simulink model "DOE_MODEL_4D"  (R2017a)
settings: Solver=VariableStepAuto  StartTime=0.0  StopTime=100  RelTol=1e-3
libraries: simulink x2
settings Model: Creator=HP  LastModifiedBy=jianx

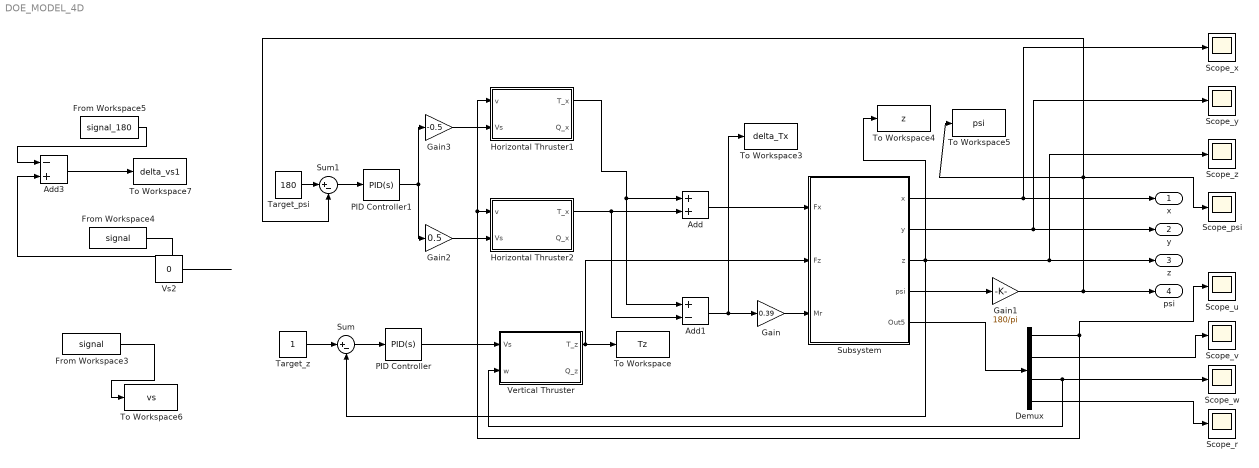
== system DOE_MODEL_4D ==
  Add : Sum
  Add1 : Sum  Inputs=+-
  Add3 : Sum  Inputs=-+
  Demux : Demux
  From Workspace3 : FromWorkspace  VariableName=signal  OutputAfterFinalValue=Setting to zero
  From Workspace4 : FromWorkspace  VariableName=signal  OutputAfterFinalValue=Setting to zero
  From Workspace5 : FromWorkspace  VariableName=signal_180  OutputAfterFinalValue=Setting to zero
  Gain : Gain  Gain=0.39
  Gain1 : Gain  Gain=180/pi
  Gain2 : Gain  Gain=0.5
  Gain3 : Gain  Gain=-0.5
  Horizontal Thruster1 : Subsystem
  Horizontal Thruster2 : Subsystem
  PID Controller : simulink/Continuous/PID Controller  Controller=PID  TimeDomain=Continuous-time  SampleTime=-1  IntegratorMethod=Forward Euler  FilterMethod=Forward Euler  Form=Parallel  UseFilter=on  ControllerParametersSource=internal  P=200  I=11.6  D=872.4  N=100  InitialConditionSource=internal  InitialConditionForIntegrator=0  InitialConditionForFilter=0  ExternalReset=none  LimitOutput=off  UpperSaturationLimit=inf  LowerSaturationLimit=-inf  LinearizeAsGain=on  AntiWindupMode=none  Kb=1  TrackingMode=off  Kt=1  PParamMin=[]  PParamMax=[]  IParamMin=[]  IParamMax=[]  DParamMin=[]  DParamMax=[]  NParamMin=[]  NParamMax=[]  KbParamMin=[]  KbParamMax=[]  KtParamMin=[]  KtParamMax=[]  POutMin=[]  POutMax=[]  IOutMin=[]  IOutMax=[]  DOutMin=[]  DOutMax=[]  NOutMin=[]  NOutMax=[]  KbOutMin=[]  KbOutMax=[]  KtOutMin=[]  KtOutMax=[]  IntegratorOutMin=[]  IntegratorOutMax=[]  FilterOutMin=[]  FilterOutMax=[]  SumOutMin=[]  SumOutMax=[]  SumI1OutMin=[]  SumI1OutMax=[]  SumI2OutMin=[]  SumI2OutMax=[]  SumI3OutMin=[]  SumI3OutMax=[]  SumDOutMin=[]  SumDOutMax=[]  SaturationOutMin=[]  SaturationOutMax=[]  IntegratorContinuousStateAttributes=''  IntegratorStateMustResolveToSignalObject=off  IntegratorRTWStateStorageClass=Auto  FilterContinuousStateAttributes=''  FilterStateMustResolveToSignalObject=off  FilterRTWStateStorageClass=Auto  DifferentiatorICPrevScaledInput=0  DifferentiatorOutMin=[]  DifferentiatorOutMax=[]  InitialConditionSetting=State (most efficient)
  PID Controller1 : simulink/Continuous/PID Controller  Controller=PID  TimeDomain=Continuous-time  SampleTime=-1  IntegratorMethod=Forward Euler  FilterMethod=Forward Euler  Form=Parallel  UseFilter=on  ControllerParametersSource=internal  P=-0.57  I=-0.021  D=-0.918  N=100  InitialConditionSource=internal  InitialConditionForIntegrator=0  InitialConditionForFilter=0  ExternalReset=none  LimitOutput=off  UpperSaturationLimit=inf  LowerSaturationLimit=-inf  LinearizeAsGain=on  AntiWindupMode=none  Kb=1  TrackingMode=off  Kt=1  PParamMin=[]  PParamMax=[]  IParamMin=[]  IParamMax=[]  DParamMin=[]  DParamMax=[]  NParamMin=[]  NParamMax=[]  KbParamMin=[]  KbParamMax=[]  KtParamMin=[]  KtParamMax=[]  POutMin=[]  POutMax=[]  IOutMin=[]  IOutMax=[]  DOutMin=[]  DOutMax=[]  NOutMin=[]  NOutMax=[]  KbOutMin=[]  KbOutMax=[]  KtOutMin=[]  KtOutMax=[]  IntegratorOutMin=[]  IntegratorOutMax=[]  FilterOutMin=[]  FilterOutMax=[]  SumOutMin=[]  SumOutMax=[]  SumI1OutMin=[]  SumI1OutMax=[]  SumI2OutMin=[]  SumI2OutMax=[]  SumI3OutMin=[]  SumI3OutMax=[]  SumDOutMin=[]  SumDOutMax=[]  SaturationOutMin=[]  SaturationOutMax=[]  IntegratorContinuousStateAttributes=''  IntegratorStateMustResolveToSignalObject=off  IntegratorRTWStateStorageClass=Auto  FilterContinuousStateAttributes=''  FilterStateMustResolveToSignalObject=off  FilterRTWStateStorageClass=Auto  DifferentiatorICPrevScaledInput=0  DifferentiatorOutMin=[]  DifferentiatorOutMax=[]  InitialConditionSetting=State (most efficient)
  Scope_psi : Scope
  Scope_r : Scope
  Scope_u : Scope
  Scope_v : Scope
  Scope_w : Scope
  Scope_x : Scope
  Scope_y : Scope
  Scope_z : Scope
  Subsystem : Subsystem
  Sum : Sum  Inputs=|+-
  Sum1 : Sum  Inputs=|+-
  Target_psi : Constant  Value=180
  Target_z : Constant
  To Workspace : ToWorkspace  VariableName=Tz  SampleTime=[0.002,0]
  To Workspace3 : ToWorkspace  VariableName=delta_Tx  SampleTime=[0.002,0]
  To Workspace4 : ToWorkspace  VariableName=z  SampleTime=[0.002,0]
  To Workspace5 : ToWorkspace  VariableName=psi  SampleTime=[0.002,0]
  To Workspace6 : ToWorkspace  VariableName=vs  SampleTime=0.002
      settings: Save2DSignal=2-D array (concatenate along first dimension)
  To Workspace7 : ToWorkspace  VariableName=delta_vs1  SampleTime=0.002
      settings: Save2DSignal=2-D array (concatenate along first dimension)
  "Vertical Thruster " : Subsystem
  Vs2 : Constant  Value=0
  x : Outport
  y : Outport  Port=2
  z : Outport  Port=3
  psi : Outport  Port=4
  wires:
  Add/1 -> Subsystem/1(Fx)
  "Vertical Thruster "/1(T_z) -> Subsystem/2(Fz), To Workspace/1
  Add1/1 -> To Workspace3/1, Gain/1
  Subsystem/1(x) -> Scope_x/1, x/1
  Subsystem/2(y) -> y/1, Scope_y/1
  Subsystem/4(psi) -> Gain1/1
  Subsystem/3(z) -> Sum/2, To Workspace4/1, z/1, Scope_z/1
  Subsystem/5(Out5) -> Demux/1
  Demux/3 -> Scope_w/1, "Vertical Thruster "/2(w)
  Demux/1 -> Horizontal Thruster1/1(v), Horizontal Thruster2/1(v), Scope_u/1
  Horizontal Thruster1/1(T_x) -> Add1/1, Add/1
  Horizontal Thruster2/1(T_x) -> Add1/2, Add/2
  Gain/1 -> Subsystem/3(Mr)
  Demux/2 -> Scope_v/1
  Gain1/1 -> Sum1/2, To Workspace5/1, Scope_psi/1, psi/1
  Demux/4 -> Scope_r/1
  From Workspace3/1 -> To Workspace6/1
  From Workspace5/1 -> Add3/1
  Add3/1 -> To Workspace7/1
  From Workspace4/1 -> Add3/2
  Vs2/1 -> ?
  Sum/1 -> PID Controller/1
  PID Controller1/1 -> Gain2/1, Gain3/1
  Sum1/1 -> PID Controller1/1
  Target_z/1 -> Sum/1
  Target_psi/1 -> Sum1/1
  Gain3/1 -> Horizontal Thruster1/2(Vs)
  Gain2/1 -> Horizontal Thruster2/2(Vs)
  PID Controller/1 -> "Vertical Thruster "/1(Vs)

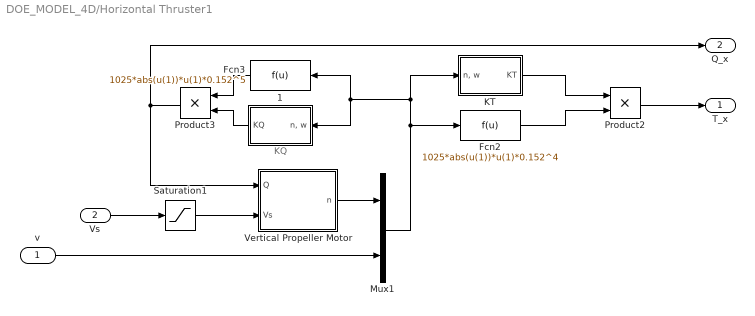
== system DOE_MODEL_4D/Horizontal Thruster1 ==
  note: KQ
  v : Inport
  Vs : Inport  Port=2
  " 1" : Subsystem
  " Vertical Propeller Motor " : Subsystem
  Fcn2 : Fcn  Expr=1025*abs(u(1))*u(1)*0.152^4
  Fcn3 : Fcn  Expr=1025*abs(u(1))*u(1)*0.152^5
  KT : Subsystem
  Mux1 : Mux  Inputs=2
  Product2 : Product
  Product3 : Product
  Saturation1 : Saturate  UpperLimit=100  LowerLimit=-100
  T_x : Outport
  Q_x : Outport  Port=2
  wires:
  Mux1/1 -> KT/1("n, w"), " 1"/1("n, w"), Fcn3/1, Fcn2/1
  Fcn3/1 -> Product3/1
  Product3/1 -> " Vertical Propeller Motor "/1("Q "), Q_x/1
  v/1 -> Mux1/2
  Fcn2/1 -> Product2/2
  " Vertical Propeller Motor "/1(n) -> Mux1/1
  KT/1(KT) -> Product2/1
  " 1"/1(KQ) -> Product3/2
  Saturation1/1 -> " Vertical Propeller Motor "/2(Vs)
  Vs/1 -> Saturation1/1
  Product2/1 -> T_x/1

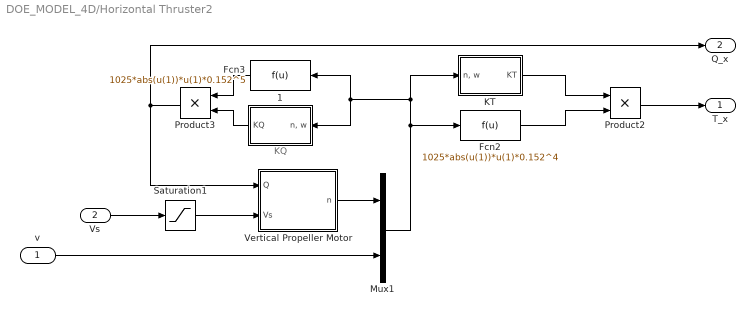
== system DOE_MODEL_4D/Horizontal Thruster2 ==
  note: KQ
  v : Inport
  Vs : Inport  Port=2
  " 1" : Subsystem
  " Vertical Propeller Motor " : Subsystem
  Fcn2 : Fcn  Expr=1025*abs(u(1))*u(1)*0.152^4
  Fcn3 : Fcn  Expr=1025*abs(u(1))*u(1)*0.152^5
  KT : Subsystem
  Mux1 : Mux  Inputs=2
  Product2 : Product
  Product3 : Product
  Saturation1 : Saturate  UpperLimit=100  LowerLimit=-100
  T_x : Outport
  Q_x : Outport  Port=2
  wires:
  Mux1/1 -> KT/1("n, w"), " 1"/1("n, w"), Fcn3/1, Fcn2/1
  Fcn3/1 -> Product3/1
  Product3/1 -> " Vertical Propeller Motor "/1("Q "), Q_x/1
  v/1 -> Mux1/2
  Fcn2/1 -> Product2/2
  " Vertical Propeller Motor "/1(n) -> Mux1/1
  KT/1(KT) -> Product2/1
  " 1"/1(KQ) -> Product3/2
  Saturation1/1 -> " Vertical Propeller Motor "/2(Vs)
  Vs/1 -> Saturation1/1
  Product2/1 -> T_x/1

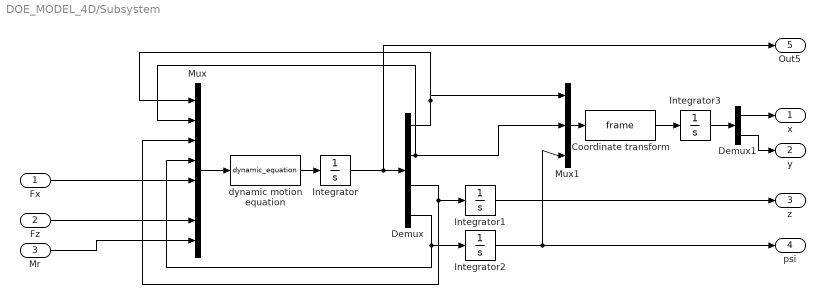
== system DOE_MODEL_4D/Subsystem ==
  Fx : Inport
  Fz : Inport  Port=2
  Mr : Inport  Port=3
  "Coordinate transform " : MATLABFcn  MATLABFcn=frame  OutputDimensions=2
  Demux : Demux
  Demux1 : Demux  Outputs=2
  Integrator{,1..3} (4 alike) : Integrator
  Mux : Mux  Inputs=8
  Mux1 : Mux  Inputs=3
  "dynamic motion equation " : MATLABFcn  MATLABFcn=dynamic_equation  OutputDimensions=4
  x : Outport
  y : Outport  Port=2
  z : Outport  Port=3
  psi : Outport  Port=4
  Out5 : Outport  Port=5
  wires:
  Fz/1 -> Mux/7
  Demux/1 -> Mux1/1, Mux/1
  Mr/1 -> Mux/8
  Integrator/1 -> Out5/1, Demux/1
  Demux/2 -> Mux1/2, Mux/2
  Demux/4 -> Integrator2/1, Mux/4
  Mux/1 -> "dynamic motion equation "/1
  Fx/1 -> Mux/5
  "dynamic motion equation "/1 -> Integrator/1
  Demux/3 -> Integrator1/1, Mux/3
  Mux1/1 -> "Coordinate transform "/1
  Integrator2/1 -> psi/1, Mux1/3
  Integrator1/1 -> z/1
  "Coordinate transform "/1 -> Integrator3/1
  Demux1/1 -> x/1
  Demux1/2 -> y/1
  Integrator3/1 -> Demux1/1

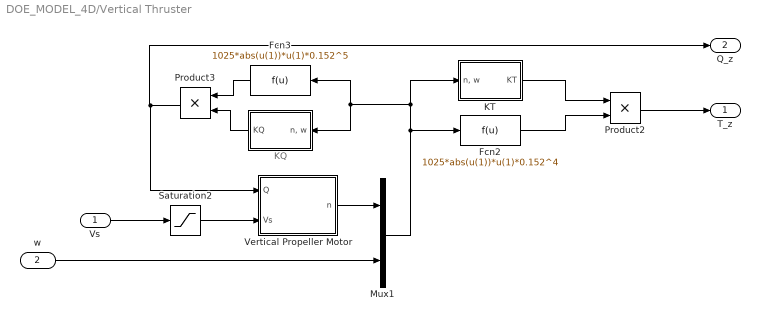
== system DOE_MODEL_4D/Vertical Thruster  ==
  note: KQ
  Vs : Inport
  w : Inport  Port=2
  " " : Subsystem
  " Vertical Propeller Motor " : Subsystem
  Fcn2 : Fcn  Expr=1025*abs(u(1))*u(1)*0.152^4
  Fcn3 : Fcn  Expr=1025*abs(u(1))*u(1)*0.152^5
  KT : Subsystem
  Mux1 : Mux  Inputs=2
  Product2 : Product
  Product3 : Product
  Saturation2 : Saturate  UpperLimit=100  LowerLimit=-100
  T_z : Outport
  Q_z : Outport  Port=2
  wires:
  Mux1/1 -> KT/1("n, w"), " "/1("n, w"), Fcn3/1, Fcn2/1
  Product2/1 -> T_z/1
  Fcn3/1 -> Product3/1
  Product3/1 -> " Vertical Propeller Motor "/1("Q "), Q_z/1
  w/1 -> Mux1/2
  Fcn2/1 -> Product2/2
  " Vertical Propeller Motor "/1(n) -> Mux1/1
  KT/1(KT) -> Product2/1
  " "/1(KQ) -> Product3/2
  Saturation2/1 -> " Vertical Propeller Motor "/2(Vs)
  Vs/1 -> Saturation2/1

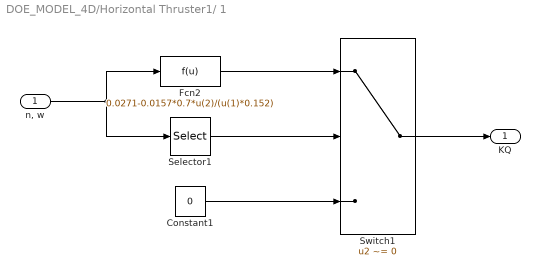
== system DOE_MODEL_4D/Horizontal Thruster1/ 1 ==
  "n, w" : Inport
  Constant1 : Constant  Value=0
  Fcn2 : Fcn  Expr=0.0271-0.0157*0.7*u(2)/(u(1)*0.152)
  Selector1 : Selector  InputPortWidth=2  IndexOptions=Index vector (dialog)  Indices=[ 1 ]  OutputSizes=1
  Switch1 : Switch  Criteria=u2 ~= 0
  KQ : Outport
  wires:
  Constant1/1 -> Switch1/3
  Switch1/1 -> KQ/1
  Fcn2/1 -> Switch1/1
  "n, w"/1 -> Fcn2/1, Selector1/1
  Selector1/1 -> Switch1/2

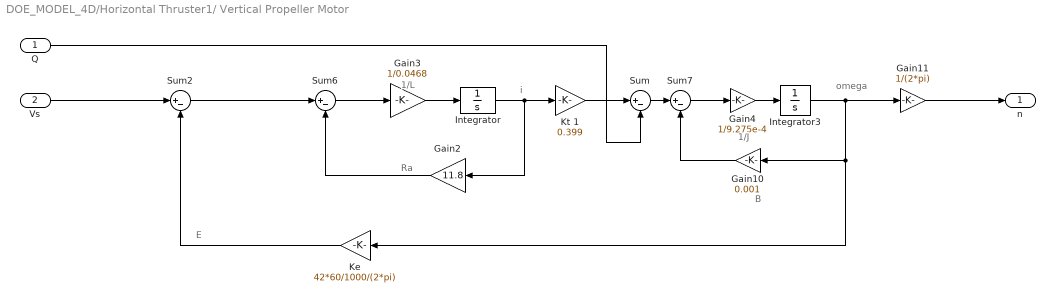
== system DOE_MODEL_4D/Horizontal Thruster1/ Vertical Propeller Motor  ==
  note: Ra
  note: i
  note: 1/J
  note: 1/L
  note: B
  note: omega
  note: E
  "Q " : Inport
  Vs : Inport  Port=2
  Gain10 : Gain  Gain=0.001  SaturateOnIntegerOverflow=on  OutDataTypeStr=Inherit: Same as input  ParamDataTypeStr=Inherit: Same as input
  Gain11 : Gain  Gain=1/(2*pi)  SaturateOnIntegerOverflow=on  OutDataTypeStr=Inherit: Same as input  ParamDataTypeStr=Inherit: Same as input
  Gain2 : Gain  Gain=11.8  OutDataTypeStr=Inherit: Same as input  ParamDataTypeStr=Inherit: Same as input
  Gain3 : Gain  Gain=1/0.0468  OutDataTypeStr=Inherit: Same as input  ParamDataTypeStr=Inherit: Same as input
  Gain4 : Gain  Gain=1/9.275e-4  SaturateOnIntegerOverflow=on  OutDataTypeStr=Inherit: Same as input  ParamDataTypeStr=Inherit: Same as input
  Integrator : Integrator
  Integrator3 : Integrator
  Ke : Gain  Gain=42*60/1000/(2*pi)
  Kt 1 : Gain  Gain=0.399
  Sum : Sum  Inputs=|+-
  Sum2 : Sum  Inputs=|+-  SaturateOnIntegerOverflow=on  InputSameDT=on  OutDataTypeStr=Inherit: Same as first input
  Sum6 : Sum  Inputs=|+-  SaturateOnIntegerOverflow=on  InputSameDT=on  OutDataTypeStr=Inherit: Same as first input
  Sum7 : Sum  Inputs=|+-  SaturateOnIntegerOverflow=on  InputSameDT=on  OutDataTypeStr=Inherit: Same as first input
  n : Outport
  wires:
  "Q "/1 -> Sum/2
  Kt 1/1 -> Sum/1
  Vs/1 -> Sum2/1
  Sum/1 -> Sum7/1
  Sum7/1 -> Gain4/1
  Gain4/1 -> Integrator3/1
  Integrator3/1 -> Ke/1, Gain10/1, Gain11/1
  Gain10/1 -> Sum7/2
  Sum2/1 -> Sum6/1
  Gain3/1 -> Integrator/1
  Gain2/1 -> Sum6/2
  Sum6/1 -> Gain3/1
  Integrator/1 -> Gain2/1, Kt 1/1
  Ke/1 -> Sum2/2
  Gain11/1 -> n/1

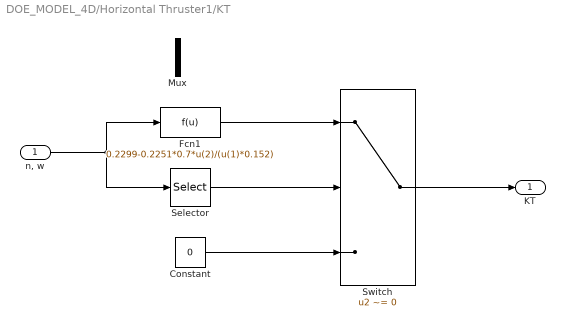
== system DOE_MODEL_4D/Horizontal Thruster1/KT ==
  "n, w" : Inport
  Constant : Constant  Value=0
  Fcn1 : Fcn  Expr=0.2299-0.2251*0.7*u(2)/(u(1)*0.152)
  Mux : Mux  Inputs=2
  Selector : Selector  InputPortWidth=2  IndexOptions=Index vector (dialog)  Indices=[ 1 ]  OutputSizes=1
  Switch : Switch  Criteria=u2 ~= 0
  KT : Outport
  wires:
  Switch/1 -> KT/1
  Constant/1 -> Switch/3
  Fcn1/1 -> Switch/1
  Selector/1 -> Switch/2
  "n, w"/1 -> Fcn1/1, Selector/1

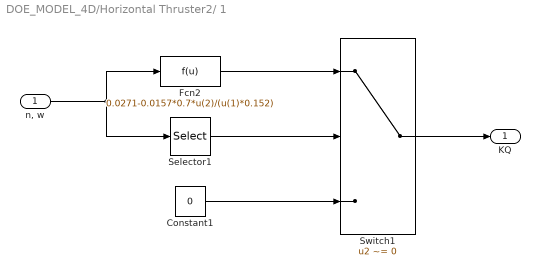
== system DOE_MODEL_4D/Horizontal Thruster2/ 1 ==
  "n, w" : Inport
  Constant1 : Constant  Value=0
  Fcn2 : Fcn  Expr=0.0271-0.0157*0.7*u(2)/(u(1)*0.152)
  Selector1 : Selector  InputPortWidth=2  IndexOptions=Index vector (dialog)  Indices=[ 1 ]  OutputSizes=1
  Switch1 : Switch  Criteria=u2 ~= 0
  KQ : Outport
  wires:
  Constant1/1 -> Switch1/3
  Switch1/1 -> KQ/1
  Fcn2/1 -> Switch1/1
  "n, w"/1 -> Fcn2/1, Selector1/1
  Selector1/1 -> Switch1/2

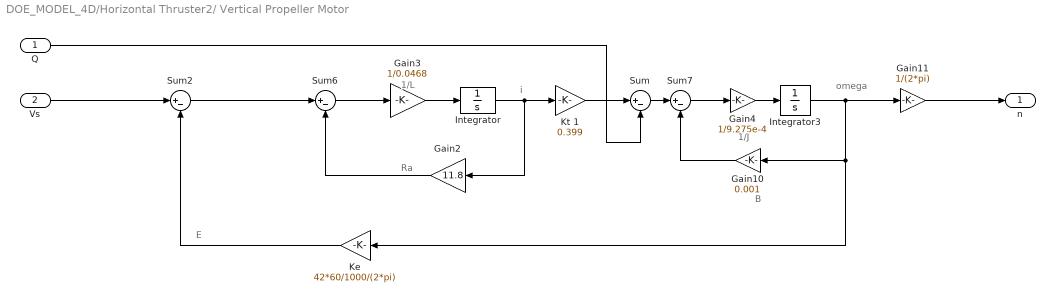
== system DOE_MODEL_4D/Horizontal Thruster2/ Vertical Propeller Motor  ==
  note: Ra
  note: i
  note: 1/J
  note: 1/L
  note: B
  note: omega
  note: E
  "Q " : Inport
  Vs : Inport  Port=2
  Gain10 : Gain  Gain=0.001  SaturateOnIntegerOverflow=on  OutDataTypeStr=Inherit: Same as input  ParamDataTypeStr=Inherit: Same as input
  Gain11 : Gain  Gain=1/(2*pi)  SaturateOnIntegerOverflow=on  OutDataTypeStr=Inherit: Same as input  ParamDataTypeStr=Inherit: Same as input
  Gain2 : Gain  Gain=11.8  OutDataTypeStr=Inherit: Same as input  ParamDataTypeStr=Inherit: Same as input
  Gain3 : Gain  Gain=1/0.0468  OutDataTypeStr=Inherit: Same as input  ParamDataTypeStr=Inherit: Same as input
  Gain4 : Gain  Gain=1/9.275e-4  SaturateOnIntegerOverflow=on  OutDataTypeStr=Inherit: Same as input  ParamDataTypeStr=Inherit: Same as input
  Integrator : Integrator
  Integrator3 : Integrator
  Ke : Gain  Gain=42*60/1000/(2*pi)
  Kt 1 : Gain  Gain=0.399
  Sum : Sum  Inputs=|+-
  Sum2 : Sum  Inputs=|+-  SaturateOnIntegerOverflow=on  InputSameDT=on  OutDataTypeStr=Inherit: Same as first input
  Sum6 : Sum  Inputs=|+-  SaturateOnIntegerOverflow=on  InputSameDT=on  OutDataTypeStr=Inherit: Same as first input
  Sum7 : Sum  Inputs=|+-  SaturateOnIntegerOverflow=on  InputSameDT=on  OutDataTypeStr=Inherit: Same as first input
  n : Outport
  wires:
  "Q "/1 -> Sum/2
  Kt 1/1 -> Sum/1
  Vs/1 -> Sum2/1
  Sum/1 -> Sum7/1
  Sum7/1 -> Gain4/1
  Gain4/1 -> Integrator3/1
  Integrator3/1 -> Ke/1, Gain10/1, Gain11/1
  Gain10/1 -> Sum7/2
  Sum2/1 -> Sum6/1
  Gain3/1 -> Integrator/1
  Gain2/1 -> Sum6/2
  Sum6/1 -> Gain3/1
  Integrator/1 -> Gain2/1, Kt 1/1
  Ke/1 -> Sum2/2
  Gain11/1 -> n/1

== system DOE_MODEL_4D/Horizontal Thruster2/KT ==
  "n, w" : Inport
  Subsystem : Subsystem
  KT : Outport
  wires:
  "n, w"/1 -> Subsystem/1("n, w")
  Subsystem/1(KT) -> KT/1

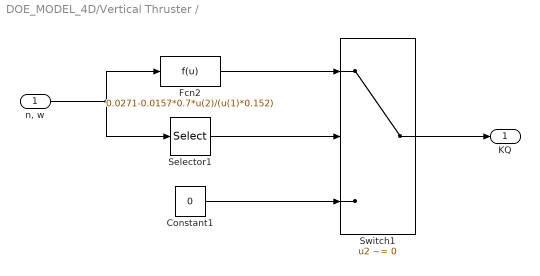
== system DOE_MODEL_4D/Vertical Thruster /  ==
  "n, w" : Inport
  Constant1 : Constant  Value=0
  Fcn2 : Fcn  Expr=0.0271-0.0157*0.7*u(2)/(u(1)*0.152)
  Selector1 : Selector  InputPortWidth=2  IndexOptions=Index vector (dialog)  Indices=[ 1 ]  OutputSizes=1
  Switch1 : Switch  Criteria=u2 ~= 0
  KQ : Outport
  wires:
  Constant1/1 -> Switch1/3
  Switch1/1 -> KQ/1
  Fcn2/1 -> Switch1/1
  "n, w"/1 -> Fcn2/1, Selector1/1
  Selector1/1 -> Switch1/2

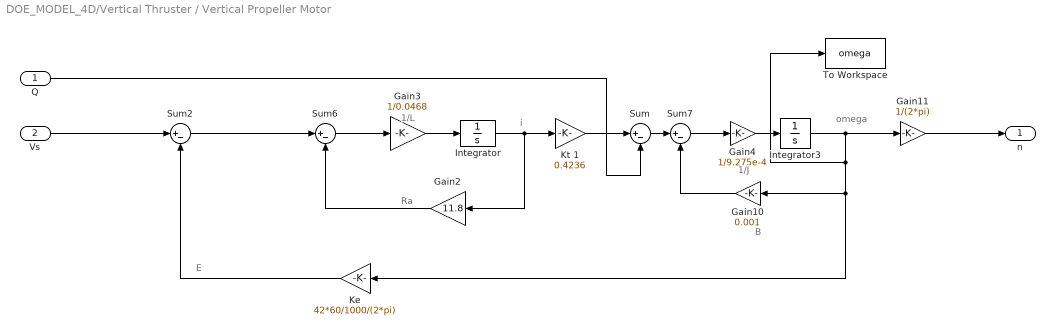
== system DOE_MODEL_4D/Vertical Thruster / Vertical Propeller Motor  ==
  note: Ra
  note: i
  note: 1/J
  note: 1/L
  note: B
  note: omega
  note: E
  "Q " : Inport
  Vs : Inport  Port=2
  Gain10 : Gain  Gain=0.001  SaturateOnIntegerOverflow=on  OutDataTypeStr=Inherit: Same as input  ParamDataTypeStr=Inherit: Same as input
  Gain11 : Gain  Gain=1/(2*pi)  SaturateOnIntegerOverflow=on  OutDataTypeStr=Inherit: Same as input  ParamDataTypeStr=Inherit: Same as input
  Gain2 : Gain  Gain=11.8  OutDataTypeStr=Inherit: Same as input  ParamDataTypeStr=Inherit: Same as input
  Gain3 : Gain  Gain=1/0.0468  OutDataTypeStr=Inherit: Same as input  ParamDataTypeStr=Inherit: Same as input
  Gain4 : Gain  Gain=1/9.275e-4  SaturateOnIntegerOverflow=on  OutDataTypeStr=Inherit: Same as input  ParamDataTypeStr=Inherit: Same as input
  Integrator : Integrator
  Integrator3 : Integrator
  Ke : Gain  Gain=42*60/1000/(2*pi)
  Kt 1 : Gain  Gain=0.4236
  Sum : Sum  Inputs=|+-
  Sum2 : Sum  Inputs=|+-  SaturateOnIntegerOverflow=on  InputSameDT=on  OutDataTypeStr=Inherit: Same as first input
  Sum6 : Sum  Inputs=|+-  SaturateOnIntegerOverflow=on  InputSameDT=on  OutDataTypeStr=Inherit: Same as first input
  Sum7 : Sum  Inputs=|+-  SaturateOnIntegerOverflow=on  InputSameDT=on  OutDataTypeStr=Inherit: Same as first input
  To Workspace : ToWorkspace  VariableName=omega  SampleTime=0.002
      settings: Save2DSignal=2-D array (concatenate along first dimension)
  n : Outport
  wires:
  "Q "/1 -> Sum/2
  Kt 1/1 -> Sum/1
  Vs/1 -> Sum2/1
  Sum/1 -> Sum7/1
  Sum7/1 -> Gain4/1
  Gain4/1 -> Integrator3/1
  Integrator3/1 -> To Workspace/1, Ke/1, Gain10/1, Gain11/1
  Gain10/1 -> Sum7/2
  Sum2/1 -> Sum6/1
  Gain3/1 -> Integrator/1
  Gain2/1 -> Sum6/2
  Sum6/1 -> Gain3/1
  Integrator/1 -> Gain2/1, Kt 1/1
  Ke/1 -> Sum2/2
  Gain11/1 -> n/1

== system DOE_MODEL_4D/Vertical Thruster /KT ==
  "n, w" : Inport
  Constant : Constant  Value=0
  Fcn1 : Fcn  Expr=0.2299-0.2251*0.7*u(2)/(u(1)*0.152)
  Selector : Selector  InputPortWidth=2  IndexOptions=Index vector (dialog)  Indices=[ 1 ]  OutputSizes=1
  Switch : Switch  Criteria=u2 ~= 0
  KT : Outport
  wires:
  Constant/1 -> Switch/3
  Switch/1 -> KT/1
  Fcn1/1 -> Switch/1
  "n, w"/1 -> Fcn1/1, Selector/1
  Selector/1 -> Switch/2

== system DOE_MODEL_4D/Horizontal Thruster2/KT/Subsystem ==
  "n, w" : Inport
  Constant : Constant  Value=0
  Fcn1 : Fcn  Expr=0.2299-0.2251*0.7*u(2)/(u(1)*0.152)
  Selector : Selector  InputPortWidth=2  IndexOptions=Index vector (dialog)  Indices=[ 1 ]  OutputSizes=1
  Switch : Switch  Criteria=u2 ~= 0
  KT : Outport
  wires:
  "n, w"/1 -> Fcn1/1, Selector/1
  Selector/1 -> Switch/2
  Fcn1/1 -> Switch/1
  Switch/1 -> KT/1
  Constant/1 -> Switch/3
